simulink model "Model_0_no_storage"  (R2019a)
settings: Solver=FixedStepAuto  StartTime=0.0  StopTime=8760  FixedStep=1  RelTol=1e-3
settings Model: Creator=senja  LastModifiedBy=senja

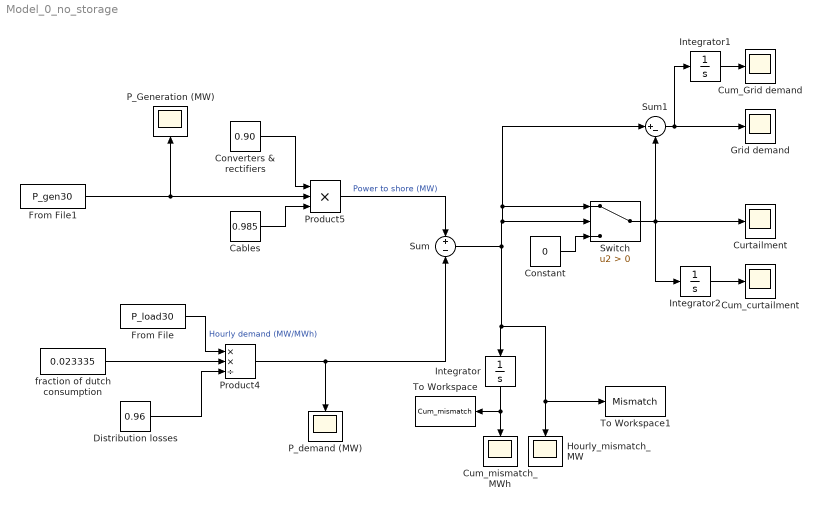
== system Model_0_no_storage ==
  Cables : Constant  Value=0.985
  Constant : Constant  Value=0
  Converters & rectifiers : Constant  Value=0.90
  Cum_Grid demand : Scope
  Cum_curtailment : Scope
  Cum_mismatch_MWh : Scope
  Curtailment : Scope
  Distribution losses : Constant  Value=0.96
  From File : FromFile  FileName=P_load30  SampleTime=0
  From File1 : FromFile  FileName=P_gen30  SampleTime=0
  Grid demand : Scope
  Hourly_mismatch_MW : Scope
  Integrator : Integrator
  Integrator1 : Integrator
  Integrator2 : Integrator
  P_Generation (MW) : Scope
  P_demand (MW) : Scope
  Product4 : Product  Inputs=**/
  Product5 : Product  Inputs=3
  Sum : Sum  Inputs=+|-
  Sum1 : Sum  Inputs=|+-
  Switch : Switch  Criteria=u2 > Threshold
  To Workspace : ToWorkspace  VariableName=Cum_mismatch  SampleTime=-1
  To Workspace1 : ToWorkspace  VariableName=Mismatch  SampleTime=-1
  fraction of dutch consumption : Constant  Value=0.023335
  wires:
  From File/1 -> Product4/1  "Hourly demand (MW/MWh)"
  fraction of dutch consumption/1 -> Product4/2
  Distribution losses/1 -> Product4/3
  Cables/1 -> Product5/3
  Converters & rectifiers/1 -> Product5/1
  Product5/1 -> Sum/1  "Power to shore (MW)"
  Product4/1 -> Sum/2, P_demand (MW)/1
  From File1/1 -> P_Generation (MW)/1, Product5/2
  Sum/1 -> Integrator/1, To Workspace1/1, Hourly_mismatch_MW/1, Sum1/1, Switch/1, Switch/2
  Integrator/1 -> To Workspace/1, Cum_mismatch_MWh/1
  Switch/1 -> Integrator2/1, Sum1/2, Curtailment/1
  Constant/1 -> Switch/3
  Sum1/1 -> Integrator1/1, Grid demand/1
  Integrator1/1 -> Cum_Grid demand/1
  Integrator2/1 -> Cum_curtailment/1
